simulink model "train_tracker"  (Simulink 7.9)
settings: Solver=ode3  StartTime=0.0  StopTime=10  FixedStep=0.001  RelTol=1e-3
settings Model: Creator=quchao  LastModifiedBy=quchao

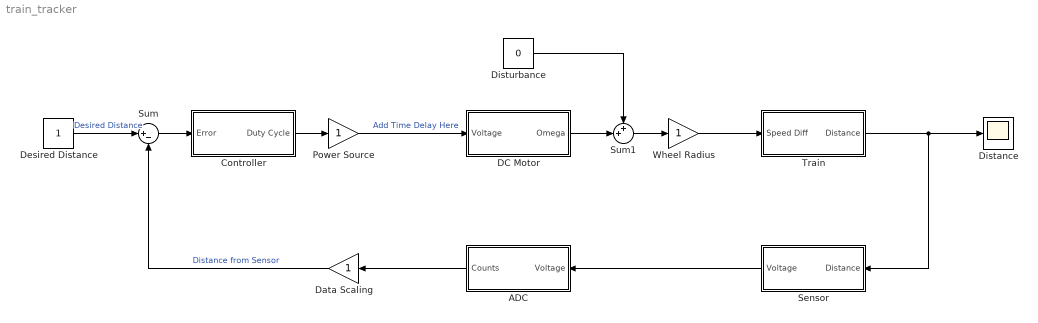
== system train_tracker ==
  ADC : Subsystem
  Controller : Subsystem
  DC Motor : Subsystem
  Data Scaling : Gain
  Desired Distance : Constant
  Distance : Scope
      settings: TimeRange=10  YMin=1.4  YMax=2
  Disturbance : Constant  Value=0
  Power Source : Gain
  Sensor : Subsystem
  Sum : Sum  Inputs=|+-
  Sum1 : Sum  Inputs=++|
  Train : Subsystem
  Wheel Radius : Gain
  wires:
  Desired Distance/1 -> Sum/1  "Desired Distance"
  Sum/1 -> Controller/1(Error)
  Controller/1(Duty Cycle) -> Power Source/1
  Power Source/1 -> DC Motor/1(Voltage)  "Add Time Delay Here"
  DC Motor/1(Omega) -> Sum1/2
  Sum1/1 -> Wheel Radius/1
  Wheel Radius/1 -> Train/1(Speed Diff)
  Disturbance/1 -> Sum1/1
  Sensor/1(Voltage) -> ADC/1(Voltage)
  ADC/1(Counts) -> Data Scaling/1
  Data Scaling/1 -> Sum/2  "Distance from Sensor"
  Train/1(Distance) -> Distance/1, Sensor/1(Distance)

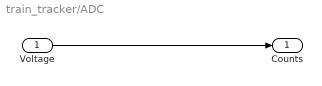
== system train_tracker/ADC ==
  Voltage : Inport
  Counts : Outport
  wires:
  Voltage/1 -> Counts/1

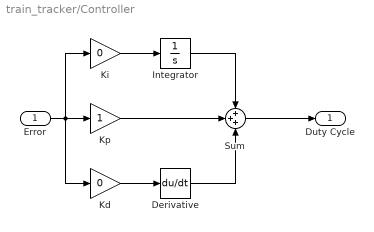
== system train_tracker/Controller ==
  Error : Inport
  Derivative : Derivative
  Integrator : Integrator
  Kd : Gain  Gain=0
  Ki : Gain  Gain=0
  Kp : Gain
  Sum : Sum  Inputs=+++
  Duty Cycle : Outport
  wires:
  Error/1 -> Kp/1, Kd/1, Ki/1
  Kp/1 -> Sum/2
  Kd/1 -> Derivative/1
  Derivative/1 -> Sum/3
  Ki/1 -> Integrator/1
  Integrator/1 -> Sum/1
  Sum/1 -> Duty Cycle/1

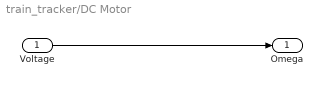
== system train_tracker/DC Motor ==
  Voltage : Inport
  Omega : Outport
  wires:
  Voltage/1 -> Omega/1

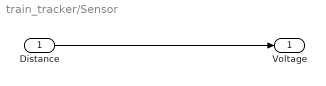
== system train_tracker/Sensor ==
  Distance : Inport
  Voltage : Outport
  wires:
  Distance/1 -> Voltage/1

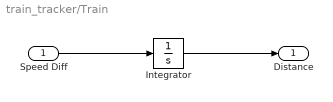
== system train_tracker/Train ==
  Speed Diff : Inport
  Integrator : Integrator  InitialCondition=2
  Distance : Outport
  wires:
  Speed Diff/1 -> Integrator/1
  Integrator/1 -> Distance/1
